simulink model "model_2018b_impact"  (R2019a)
settings: Solver=VariableStepAuto  StartTime=0.0  StopTime=0.1  RelTol=1e-3
settings Model: EnablePacing=on  PacingRate=1000  Creator=akulkarni  LastModifiedBy=akulkarni
settings DataIOCC: InspectSignalLogs=on
settings DebuggingCC: ArithmeticOperatorsInVariantConditions=warning

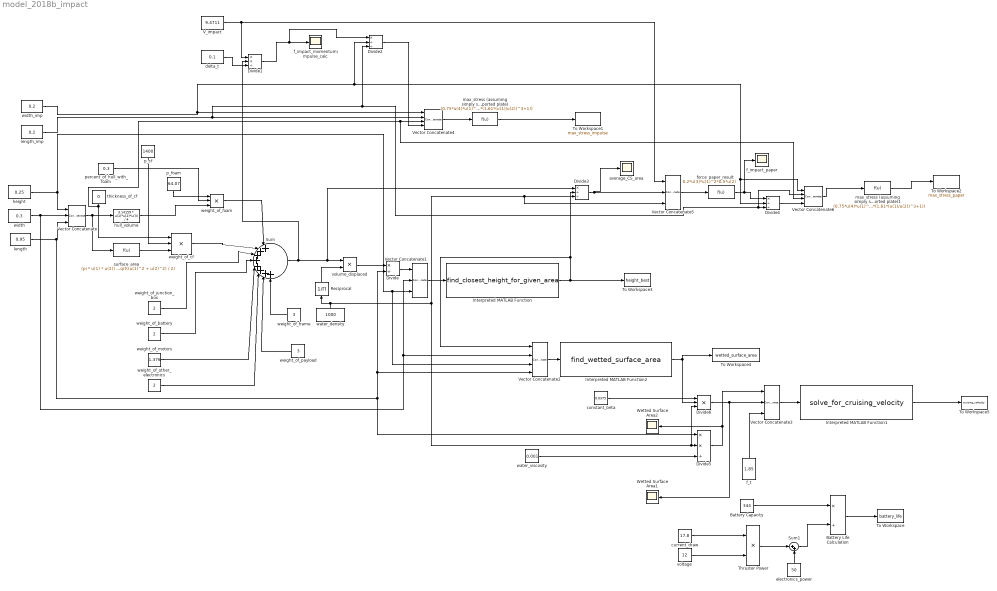
== system model_2018b_impact ==
  Battery Capacity : Constant  Value=344
  Battery Life Calculation : Product  Inputs=*/
  Divide : Product  Inputs=*/
  Divide1 : Product  Inputs=**/
  Divide2 : Product  Inputs=*//
  Divide3 : Product  Inputs=*//
  Divide4 : Product  Inputs=*//
  Divide5 : Product  Inputs=**/
  Divide6 : Product  Inputs=***
  Interpreted MATLAB Function : MATLABFcn  MATLABFcn=find_closest_height_for_given_area  OutputDimensions=1
  Interpreted MATLAB Function1 : MATLABFcn  MATLABFcn=solve_for_cruising_velocity  OutputDimensions=1
  Interpreted MATLAB Function2 : MATLABFcn  MATLABFcn=find_wetted_surface_area  OutputDimensions=1
  Reciprocal : Product  Inputs=/
  Sum : Sum  Inputs=|++++++++
  Sum1 : Sum  Inputs=|++
  Thruster Power : Product
  To Workspace : ToWorkspace  VariableName=battery_life  SampleTime=-1
  To Workspace1 : ToWorkspace  VariableName=max_stress_impulse  SampleTime=-1
  To Workspace2 : ToWorkspace  VariableName=max_stress_paper  SampleTime=-1
  To Workspace3 : ToWorkspace  VariableName=height_best  SampleTime=-1
  To Workspace4 : ToWorkspace  VariableName=wetted_surface_area  SampleTime=-1
  To Workspace5 : ToWorkspace  VariableName=cruising_velocity  SampleTime=-1
  V_impact : Constant  Value=9.4711
  Vector Concatenate{,1,3,5} (4 alike) : Concatenate  NumInputs=3
  Vector Concatenate2 : Concatenate  NumInputs=4
  Vector Concatenate4 : Concatenate  NumInputs=4
  Vector Concatenate6 : Concatenate  NumInputs=4
  Wetted Surface Area1 : Scope
  Wetted Surface Area2 : Scope
  average_CS_area : Scope
  constant_beta : Constant  Value=0.0375
  current_draw : Constant  Value=17.8
  delta_t : Constant  Value=0.1
  electronics_power : Constant  Value=50
  f_impact_momentumimpulse_calc : Scope
  f_impact_paper : Scope
  f_t : Constant  Value=1.85
  force_paper_result : Fcn  Expr=0.2*u(3)*u(1)^2*0.5*u(2)
  height : Constant  Value=0.25
  hull_volume : Fcn  Expr=3.14159 * u(1)*u(2)*u(3) / 4
  length : Constant  Value=0.95
  length_imp : Constant  Value=0.2
  max_stress (assuming simply supported plate) : Fcn  Expr=(0.75*u(4)*u(1)^2)/(u(3)^2*(1.61*(u(1)/u(2))^3+1))
  max_stress (assuming simply supported plate)1 : Fcn  Expr=(0.75*u(4)*u(1)^2)/(u(3)^2*(1.61*(u(1)/u(2))^3+1))
  p_cf : Constant  Value=1400
  p_foam : Constant  Value=64.07
  percent_of_hull_with_foam : Constant  Value=0.3
  "surface_area " : Fcn  Expr=(pi * u(1) * u(2)) / 2 + pi * u(3) * sqrt((u(1)^2 + u(2)^2) / 2)
  thickness_of_cf : Constant  Value=0
  voltage : Constant  Value=12
  volume_displaced : Product
  water_density : Constant  Value=1000
  water_viscosity : Constant  Value=0.001
  weight_of_battery : Constant  Value=2
  weight_of_cf : Product  Inputs=3
  weight_of_foam : Product  Inputs=3
  weight_of_frame : Constant  Value=3
  weight_of_junction_box : Constant  Value=2
  weight_of_motors : Constant  Value=1.376
  weight_of_other_electronics : Constant  Value=2
  weight_of_payload : Constant  Value=3
  width : Constant  Value=0.3
  width_imp : Constant  Value=0.2
  wires:
  p_foam/1 -> weight_of_foam/1
  percent_of_hull_with_foam/1 -> weight_of_foam/2
  height/1 -> Vector Concatenate/1, Vector Concatenate2/3, Vector Concatenate1/3
  length/1 -> Divide5/1, Divide/2, Vector Concatenate2/4, Vector Concatenate/3
  Vector Concatenate/1 -> "surface_area "/1, hull_volume/1
  hull_volume/1 -> weight_of_foam/3
  "surface_area "/1 -> weight_of_cf/3
  p_cf/1 -> weight_of_cf/2
  thickness_of_cf/1 -> weight_of_cf/1, Vector Concatenate6/3, Vector Concatenate4/3
  weight_of_foam/1 -> Sum/1
  weight_of_cf/1 -> Sum/2
  weight_of_junction_box/1 -> Sum/3
  weight_of_battery/1 -> Sum/4
  weight_of_motors/1 -> Sum/5
  weight_of_other_electronics/1 -> Sum/6
  Sum/1 -> Divide1/2, Divide3/1, volume_displaced/1
  water_density/1 -> Reciprocal/1, Divide6/3, Divide5/2, Vector Concatenate5/3, Divide3/3
  Reciprocal/1 -> volume_displaced/2
  volume_displaced/1 -> Divide/1
  Divide/1 -> Vector Concatenate1/1
  weight_of_frame/1 -> Sum/8
  weight_of_payload/1 -> Sum/7
  Vector Concatenate1/1 -> Interpreted MATLAB Function/1
  Interpreted MATLAB Function/1 -> To Workspace3/1, Divide3/2, Vector Concatenate2/1
  width/1 -> Vector Concatenate/2, Vector Concatenate1/2, Vector Concatenate2/2
  Vector Concatenate2/1 -> Interpreted MATLAB Function2/1
  Interpreted MATLAB Function2/1 -> Divide6/2, To Workspace4/1
  Vector Concatenate3/1 -> Interpreted MATLAB Function1/1
  f_t/1 -> Vector Concatenate3/3
  V_impact/1 -> Vector Concatenate5/1, Divide1/1
  delta_t/1 -> Divide1/3
  Divide1/1 -> Divide2/1, f_impact_momentumimpulse_calc/1
  width_imp/1 -> Vector Concatenate6/1, Divide4/2, Divide2/2, Vector Concatenate4/1
  length_imp/1 -> Vector Concatenate6/2, Divide4/3, Divide2/3, Vector Concatenate4/2
  Vector Concatenate4/1 -> max_stress (assuming simply supported plate)/1
  Divide2/1 -> Vector Concatenate4/4
  Divide3/1 -> Vector Concatenate5/2, average_CS_area/1
  Vector Concatenate5/1 -> force_paper_result/1
  Divide4/1 -> Vector Concatenate6/4
  Vector Concatenate6/1 -> max_stress (assuming simply supported plate)1/1
  force_paper_result/1 -> Divide4/1, f_impact_paper/1
  current_draw/1 -> Thruster Power/1
  voltage/1 -> Thruster Power/2
  Thruster Power/1 -> Sum1/1
  electronics_power/1 -> Sum1/2
  Sum1/1 -> Battery Life Calculation/2
  Battery Capacity/1 -> Battery Life Calculation/1
  Battery Life Calculation/1 -> To Workspace/1
  Interpreted MATLAB Function1/1 -> To Workspace5/1
  max_stress (assuming simply supported plate)1/1 -> To Workspace2/1
  max_stress (assuming simply supported plate)/1 -> To Workspace1/1
  water_viscosity/1 -> Divide5/3
  Divide5/1 -> Wetted Surface Area2/1, Vector Concatenate3/1
  constant_beta/1 -> Divide6/1
  Divide6/1 -> Wetted Surface Area1/1, Vector Concatenate3/2
